simulink model "AuE8930_G2"  (R2023a)
settings: Solver=VariableStepAuto  StartTime=0  StopTime=2474  FixedStep=0.1  RelTol=1e-3
undefined symbols (not defined in the file): Af, alpha, Battery, Cd, eff_trans, EM_Omega_Max, EM_Torque_Max, frr, Ft_r_accl, Ft_r_decl, Fuel_Cell, g, Ki, Kp, mass, r_tire, ratio_fd, rho_air
libraries: fl_lib x16, nesl_utility x13, ee_lib x8, autolibshared x1, slpidlib x1, batteryecm_lib x1
settings Model: PacingRate=1000  Creator=akilp  LastModifiedBy=amrut
settings DebuggingCC: AlgebraicLoopMsg=none  UnconnectedInputMsg=warning  UnconnectedOutputMsg=warning  UnconnectedLineMsg=warning
settings ModelReferenceCC: EnableRefExpFcnMdlSchedulingChecks=on
settings SFSimCC: CustomCodeUndefinedFunction=UseInterfaceOnly
settings RTWCC: DLArmComputeVersion=19.05

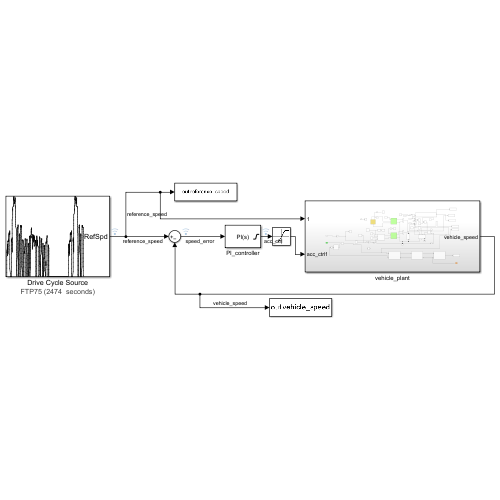
[thumbnail: Simulink's stored preview of the top-level diagram]
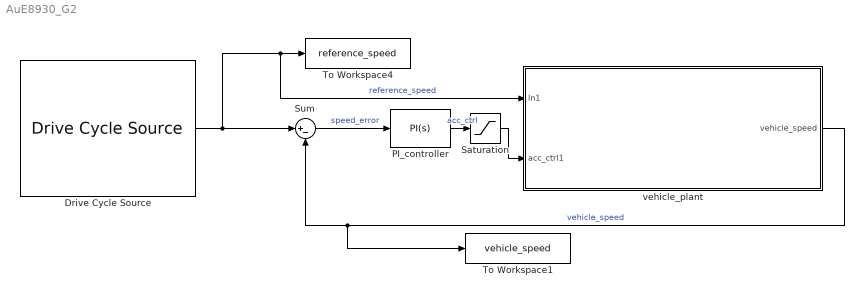
== system AuE8930_G2 ==
  Drive Cycle Source : autolibshared/Drive Cycle Source  cycleVar=FTP75  wsVar=high_trans_speed  fileVar=cycleFTP75.mat  tfinal="2474  seconds"  cycleRepeat=off  outAccPort=off  outGearPort=off  gearList=No gear data  t_wot1=5  xdot_woto=0  xdot_wot1=30  t_wot2=20  xdot_wot2=0  t_wotend=30  srcUnit=m/s  outUnit=m/s  srcAccUnit=m/s/s  outAccUnit=m/s^2  dt=0  aMode=1  faultOption=off  velBnd=2  velBndUnit=mph  inUnit=m/s  timeBnd=1  failOption=off  stopSim=off  maxFaultCnt=10  maxFaultTime=2  maxTotFaultTime=15  traceOption=off  dtTrace=1  traceWindow=10  lastDCname=FTP75  lastOutUnit=mph  lastDT=0  lastTB=1  lastSB=2  forceCalcBound=off
  "PI_controller " : slpidlib/PID Controller  Controller=PI  Form=Parallel  TimeDomain=Continuous-time  UseExternalTs=off  SampleTime=-1  IntegratorMethod=Forward Euler  FilterMethod=Forward Euler  ControllerParametersSource=internal  P=Kp  I=Ki  UseKiTs=off  D=0  N=100  UseFilter=on  TunerSelectOption=Transfer Function Based (PID Tuner App)  InitialConditionSource=internal  InitialConditionForIntegrator=0  InitialConditionForFilter=0  DifferentiatorICPrevScaledInput=0  ExternalReset=none  TrackingMode=off  Kt=1  LimitOutput=on  SatLimitsSource=internal  UpperSaturationLimit=1  LowerSaturationLimit=-1  LinearizeAsGain=on  AntiWindupMode=back-calculation  Kb=1  LimitIntegrator=off  UpperIntegratorSaturationLimit=inf  LowerIntegratorSaturationLimit=-inf  POutMin=[]  POutMax=[]  IOutMin=[]  IOutMax=[]  DOutMin=[]  DOutMax=[]  NOutMin=[]  NOutMax=[]  SumOutMin=[]  SumOutMax=[]  SaturationOutMin=[]  SaturationOutMax=[]  PParamMin=[]  PParamMax=[]  IParamMin=[]  IParamMax=[]  DParamMin=[]  DParamMax=[]  NParamMin=[]  NParamMax=[]  KbParamMin=[]  KbParamMax=[]  KtParamMin=[]  KtParamMax=[]  KbOutMin=[]  KbOutMax=[]  KtOutMin=[]  KtOutMax=[]  IntegratorOutMin=[]  IntegratorOutMax=[]  FilterOutMin=[]  FilterOutMax=[]  SumI1OutMin=[]  SumI1OutMax=[]  SumI2OutMin=[]  SumI2OutMax=[]  SumI3OutMin=[]  SumI3OutMax=[]  SumI4OutMin=[]  SumI4OutMax=[]  SumDOutMin=[]  SumDOutMax=[]  DifferentiatorOutMin=[]  DifferentiatorOutMax=[]  FilterDiffOutCoefMin=[]  FilterDiffOutCoefMax=[]  ReciprocalOutMin=[]  ReciprocalOutMax=[]  SumDenOutMin=[]  SumDenOutMax=[]  SumNumOutMin=[]  SumNumOutMax=[]  DivideOutMin=[]  DivideOutMax=[]  UdiffTsProdOutMin=[]  UdiffTsProdOutMax=[]  NTsProdOutMin=[]  NTsProdOutMax=[]  UintegralTsProdOutMin=[]  UintegralTsProdOutMax=[]  UngainTsProdOutMin=[]  UngainTsProdOutMax=[]  ClampingZeroOutDataTypeStr=Inherit: Inherit via back propagation  ClampingZeroOutMin=[]  ClampingZeroOutMax=[]  FilterDenConstantOutDataTypeStr=Inherit: Inherit via back propagation  FilterDenConstantOutMin=[]  FilterDenConstantOutMax=[]  PCopyOutDataTypeStr=Inherit: Inherit via back propagation  PCopyOutMin=[]  PCopyOutMax=[]  NCopyOutDataTypeStr=Inherit: Inherit via back propagation  NCopyOutMin=[]  NCopyOutMax=[]  IntegratorContinuousStateAttributes=''  IntegratorStateMustResolveToSignalObject=off  IntegratorRTWStateStorageClass=Auto  FilterContinuousStateAttributes=''  FilterStateMustResolveToSignalObject=off  FilterRTWStateStorageClass=Auto  ParallelPVariant=InternalParameters  IdealPVariant=Disabled  IVariant=InternalParameters  DVariant=Disabled  IntegratorVariant=Continuous  SatVariant=Enabled  AWVariant=BackCalculation  PCopyVariant=Disabled  TRVariant=Disabled  FdbkBlocksVariant=Forward  IdealPFdbkVariant=Disabled  SatFdbkVariant=Disabled  DerivativeFilterVariant=Disabled  NVariant=Disabled  NCopyVariant=Disabled_SignalSpec  FilterICVariant=Disabled  IntegratorICVariant=InternalICs  ExternalResetVariant=Disabled  TRSumVariant=Passthrough  SumFdbkVariant=Disabled  SumVariant=Sum_PI  TsampFilterVariant=InternalTs  TsampNgainVariant=Passthrough  TsampIntegralVariant=Disabled_SignalSpec  ExternalSaturationOutDataTypeStr=Inherit: Same as second input
  Saturation : Saturate  UpperLimit=100  LowerLimit=-100
  Sum : Sum  Inputs=|+-
  To Workspace1 : ToWorkspace  VariableName=vehicle_speed  SaveFormat=Timeseries  SampleTime=-1
  To Workspace4 : ToWorkspace  VariableName=reference_speed  SaveFormat=Timeseries  SampleTime=-1
  vehicle_plant : Subsystem
  wires:
  Sum/1 -> "PI_controller "/1  "speed_error"
  Drive Cycle Source/1 -> vehicle_plant/1(In1), To Workspace4/1, Sum/1  "reference_speed"
  vehicle_plant/1(vehicle_speed) -> To Workspace1/1, Sum/2  "vehicle_speed"
  "PI_controller "/1 -> Saturation/1  "acc_ctrl"
  Saturation/1 -> vehicle_plant/2(acc_ctrl1)

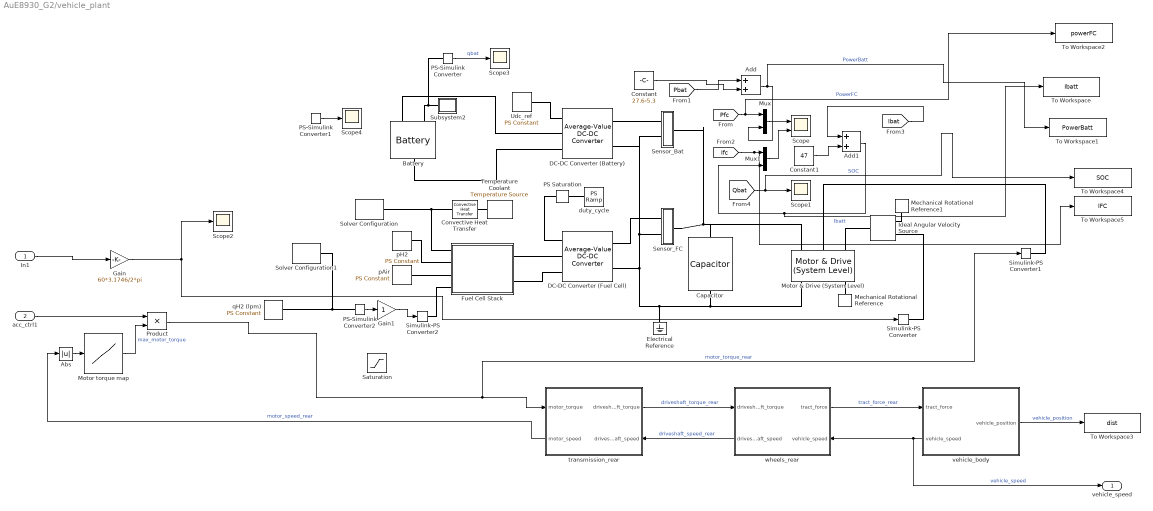
== system AuE8930_G2/vehicle_plant ==
  In1 : Inport
  acc_ctrl1 : Inport  Port=2
  Abs : Abs  SaturateOnIntegerOverflow=off
  Add : Sum
  Add1 : Sum
  Battery : batteryecm_lib/Battery  Vnom=Battery.Unom V  prm_dir=simscape.enum.battery.prm_dir.disabled  R1_dis=2 Ohm  R1_ch=2 Ohm  R1=Battery.Resistance Ohm  prm_AH=2  AH=Battery.Qnom hr*A  V1=Battery.U1 V  AH1=Battery.Q1 hr*A  prm_R2=1  R2=2000 Ohm  Tmeas=298.15 K  charge_measurement_port=simscape.enum.battery.enable.yes  prm_dyn=1  Rp1=0.005 Ohm  tau1=30 s  Rp2=0.005 Ohm  tau2=30 s  Rp3=0.005 Ohm  tau3=30 s  Rp4=0.005 Ohm  tau4=30 s  Rp5=0.005 Ohm  tau5=30 s  prm_fade=1  N_fade=100  AH_fade=45 hr*A  R1_fade=2.02 Ohm  R1_ch_fade=2.02 Ohm  V1_fade=10.35 V  prm_age=1  prm_age_OCV=1  OCV_age=0.9  SOC_age=60  Tmeas_age=298.15 K  delta_time_age_vec=[0] d  temperature_age_vec=[273] K  OCV_scaling_age=2.2134e6  OCV_offset_age=1.632e6  temp_exp_age=0.515833569 V  t_exp_age=0.75  Vnom_T2=12 V  R1_T2=2.2 Ohm  R1_T2_dis=2.2 Ohm  R1_T2_ch=2.2 Ohm  V1_T2=11.4 V  R2_T2=2200 Ohm  Rp1_T2=0.005 Ohm  tau1_T2=30 s  Rp2_T2=0.005 Ohm  tau2_T2=30 s  Rp3_T2=0.005 Ohm  tau3_T2=30 s  Rp4_T2=0.005 Ohm  tau4_T2=30 s  Rp5_T2=0.005 Ohm  tau5_T2=30 s  Tmeas2=273.15 K  thermal_port=simscape.enum.thermaleffects.omit  thermal_mass=30000 J/K  i_specify=off  i_priority=None  i=0 A  i_nominal_specify=off  i_nominal_unit=A  i_nominal_value=1  v_specify=on  v_priority=High  v=Battery.Uinit V  v_nominal_specify=off  v_nominal_unit=V  v_nominal_value=1  charge_specify=on  charge_priority=High  charge=Battery.Qnom hr*A  charge_nominal_specify=off  charge_nominal_unit=A*hr  charge_nominal_value=1  num_cycles_specify=off  num_cycles_priority=High  num_cycles=0  num_cycles_nominal_specify=off  num_cycles_nominal_unit=1  num_cycles_nominal_value=1  temperature_specify=off  temperature_priority=High  temperature=298.15 K  temperature_nominal_specify=off  temperature_nominal_unit=K  temperature_nominal_value=1
      settings: LogSimulationData=on  InternalSimscapePortConfiguration="{\"Bottom\":[],\"Left\":[{\"id\":\"p\",\"label\":\"+\",\"type\":\"foundation.electrical.electrical\"},{\"id\":\"q\",\"label\":\"q\",\"type\":\"output\"}],\"Right\":[{\"id\":\"n\",\"label\":\"-\",\"type\":\"foundation.electrical.electrical\"}],\"Top\":[]}"
  Capacitor : fl_lib/Electrical/Electrical Elements/Capacitor  c=5 mF  r=0.05 Ohm  g=0 1/Ohm  i_specify=off  i_priority=None  i=0 A  i_nominal_specify=off  i_nominal_unit=A  i_nominal_value=1  v_specify=off  v_priority=None  v=0 V  v_nominal_specify=off  v_nominal_unit=V  v_nominal_value=1  vc_specify=on  vc_priority=High  vc=500 V  vc_nominal_specify=off  vc_nominal_unit=V  vc_nominal_value=1
  Constant : Constant  Value=27.6-5.3
  Constant1 : Constant  Value=47
  Convective Heat Transfer : fl_lib/Thermal/Thermal Elements/Convective Heat Transfer  thermal_type=foundation.enum.constant_variable.constant  area=300 cm^2  heat_tr_coeff=75 W/(m^2 * K)  min_heat_tr_coeff=1e-3 W/(K*m^2)  T_specify=off  T_priority=None  T=0 K  T_nominal_specify=off  T_nominal_unit=K  T_nominal_value=1  Q_specify=off  Q_priority=None  Q=0 W  Q_nominal_specify=off  Q_nominal_unit=W  Q_nominal_value=1
  DC-DC Converter (Battery) : ee_lib/Semiconductors & Converters/Converters/Average-Value DC-DC Converter  control_option=ee.enum.converters.controlinput.voltage  converter_type=ee.enum.converters.dcdctype.boost  efficiency_option=ee.enum.converters.efficiency.constant  efficiency_fixed=100  i_vec=[0, 2, 5] A  efficiency_vec=[90, 95, 98]
      settings: LogSimulationData=on  InternalSimscapePortConfiguration="{\"Bottom\":[],\"Left\":[{\"id\":\"Vref\",\"label\":\"Vref\",\"type\":\"input\"},{\"id\":\"p1\",\"label\":\"1+\",\"type\":\"foundation.electrical.electrical\"},{\"id\":\"n1\",\"label\":\"1-\",\"type\":\"foundation.electrical.electrical\"}],\"Right\":[{\"id\":\"p2\",\"label\":\"2+\",\"type\":\"foundation.electrical.electrical\"},{\"id\":\"n2\",\"label\":\"2-\",\"type\":\"foundation.electrical.electrical\"}],\"Top\":[]}"
  DC-DC Converter (Fuel Cell) : ee_lib/Semiconductors & Converters/Converters/Average-Value DC-DC Converter  control_option=ee.enum.converters.controlinput.dutycycle  converter_type=ee.enum.converters.dcdctype.boost  efficiency_option=ee.enum.converters.efficiency.constant  efficiency_fixed=100  i_vec=[0, 2, 5] A  efficiency_vec=[90, 95, 98]
      settings: LogSimulationData=on  InternalSimscapePortConfiguration="{\"Bottom\":[],\"Left\":[{\"id\":\"DutyCycle\",\"label\":\"DutyCycle\",\"type\":\"input\"},{\"id\":\"p1\",\"label\":\"1+\",\"type\":\"foundation.electrical.electrical\"},{\"id\":\"n1\",\"label\":\"1-\",\"type\":\"foundation.electrical.electrical\"}],\"Right\":[{\"id\":\"p2\",\"label\":\"2+\",\"type\":\"foundation.electrical.electrical\"},{\"id\":\"n2\",\"label\":\"2-\",\"type\":\"foundation.electrical.electrical\"}],\"Top\":[]}"
  Electrical Reference : fl_lib/Electrical/Electrical Elements/Electrical Reference
  Fuel Cell Stack : Subsystem
  Gain : Gain  Gain=60*3.1746/2*pi
  Gain1 : Gain
  Ideal Angular Velocity Source : fl_lib/Mechanical/Mechanical Sources/Ideal Angular Velocity Source
  Mechanical Rotational Reference : fl_lib/Mechanical/Rotational Elements/Mechanical Rotational Reference
  Mechanical Rotational Reference1 : fl_lib/Mechanical/Rotational Elements/Mechanical Rotational Reference
  Motor & Drive (System Level) : ee_lib/Electromechanical/Motor & Drive (System Level)  torque_speed_param=ee.enum.electromech.envelope.torque_power  overtorque_param=ee.enum.electromech.overtorque.no  T_t=[.09, .08, .07, 0] N*m  T_t_intermittent=[.36, .32, .28, 0] N*m  T_t_2D=[.09, .09, .09; .08, .08, .08; .07, .07, .07; 0, 0, 0] N*m  T_t_intermittent_2D=[.36, .36, .36; .32, .32, .32; .28, .28, .28; 0, 0, 0] N*m  w_t=[0, 3750, 7500, 8000] rpm  vdc_t=[6, 12, 24] V  torque_max=Electric_Motor.Torque N*m  power_max=Electric_Motor.Power kW  torque_max_intermittent=0.4 N*m  power_max_intermittent=120 W  time_overtorque=30 s  time_recover=60 s  Tc=0.02 s  losses_param=1  eff=100  w_eff=3750 rpm  T_eff=0.08 N*m  Piron=0 W  Pbase=0 W  w_eff_vec=[-8000, -4000, 0, 4000, 8000] rpm  T_eff_vec=[0, .03, .06, .09] N*m  v_eff_vec=[100, 250, 400] V  losses_mat=[1.49, 1.67, 2.21, 3.1; .42, .69, 1.14, 2.03; .06, .24, .78, 1.68; .42, .69, 1.14, 2.03; 1.49, 1.67, 2.21, 3.1] W  efficiency_mat=[95, 95, 95, 95; 95, 95, 95, 95; 95, 95, 95, 95; 95, 95, 95, 95; 95, 95, 95, 95]  losses_mat_3D=ones(5, 4, 3) W  efficiency_mat_3D=95 * ones(5, 4, 3)  Res=0 Ohm  enable_fault=simscape.enum.onoff.off  fault_condition=1  fault_threshold=0.5  J=5e-6 kg*m^2  lam=1e-5 N*m/(rad/s)  speed0=0 rpm  faulted_specify=off  faulted_priority=None  faulted=0  faulted_nominal_specify=off  faulted_nominal_unit=1  faulted_nominal_value=1  torqueLimitContinuous_specify=off  torqueLimitContinuous_priority=None  torqueLimitContinuous=0 N*m  torqueLimitContinuous_nominal_specify=off  torqueLimitContinuous_nominal_unit=N*m  torqueLimitContinuous_nominal_value=1  alpha=3.93e-3 1/K  Tmeas=25 degC  Tmeas2=125 degC  losses_mat_T2=[1.49, 1.74, 2.49, 3.74; .42, .67, 1.42, 2.67; .06, .31, 1.06, 2.31; .42, .67, 1.42, 2.67; 1.49, 1.74, 2.49, 3.74] W  efficiency_mat_T2=[95, 95, 95, 95; 95, 95, 95, 95; 95, 95, 95, 95; 95, 95, 95, 95; 95, 95, 95, 95]  losses_mat_3D_T2=ones(5, 4, 3) W  efficiency_mat_3D_T2=95 * ones(5, 4, 3)  thermal_mass=100 J/K  initial_temperature=25 degC
  Motor torque map : Lookup_n-D  NumberOfTableDimensions=1  BreakpointsForDimension1=EM_Omega_Max  BreakpointsForDimension2=alpha  Table=EM_Torque_Max  ExtrapMethod=Clip  UseLastTableValue=on  InternalRulePriority=Speed  RndMeth=Simplest
  Mux : Mux  Inputs=2
  Mux1 : Mux  Inputs=2
  PS Saturation : fl_lib/Physical Signals/Nonlinear Operators/PS Saturation  upper_limit=0.95  lower_limit=0.15
  PS-Simulink Converter : nesl_utility/PS-Simulink Converter  PhysicalDomain=network_engine_domain  SubClassName=ps_output  LeftPortType=input  RightPortType=output  PseudoPeriodic=off  Frequencies=[]  VectorFormat=inherit  Unit=inherit  AffineConversion=off
  PS-Simulink Converter1 : nesl_utility/PS-Simulink Converter  PhysicalDomain=network_engine_domain  SubClassName=ps_output  LeftPortType=input  RightPortType=output  PseudoPeriodic=off  Frequencies=[]  VectorFormat=inherit  Unit=inherit  AffineConversion=off
  PS-Simulink Converter2 : nesl_utility/PS-Simulink Converter  PhysicalDomain=network_engine_domain  SubClassName=ps_output  LeftPortType=input  RightPortType=output  PseudoPeriodic=off  Frequencies=[]  VectorFormat=inherit  Unit=inherit  AffineConversion=off
  Product : Product
  Saturation : Saturate
  Scope : Scope  NumInputPorts=2
  Scope{1..4} (4 alike) : Scope
  Sensor_Bat : Subsystem
  Sensor_FC : Subsystem
  Simulink-PS Converter : nesl_utility/Simulink-PS Converter  PhysicalDomain=network_engine_domain  SubClassName=ps_input  LeftPortType=input  RightPortType=output  PseudoPeriodic=off  Frequencies=[]  NoiseDistribution=none  NoiseParameters=[]  Unit=rad/s  AffineConversion=off  FilteringAndDerivatives=filter  SimscapeFilterOrder=1  InputFilterTimeConstant=1  UdotUserProvided=0
  Simulink-PS Converter1 : nesl_utility/Simulink-PS Converter  PhysicalDomain=network_engine_domain  SubClassName=ps_input  LeftPortType=input  RightPortType=output  PseudoPeriodic=off  Frequencies=[]  NoiseDistribution=none  NoiseParameters=[]  Unit=N*m  AffineConversion=off  FilteringAndDerivatives=filter  SimscapeFilterOrder=1  InputFilterTimeConstant=1  UdotUserProvided=0
  Simulink-PS Converter2 : nesl_utility/Simulink-PS Converter  PhysicalDomain=network_engine_domain  SubClassName=ps_input  LeftPortType=input  RightPortType=output  PseudoPeriodic=off  Frequencies=[]  NoiseDistribution=none  NoiseParameters=[]  Unit=1  AffineConversion=off  FilteringAndDerivatives=provide  SimscapeFilterOrder=1  InputFilterTimeConstant=0.001  UdotUserProvided=0
  Solver Configuration : nesl_utility/Solver Configuration  PhysicalDomain=network_engine_domain  SubClassName=solver  LeftPortType=input  RightPortType=generic  Tones=[]  Harmonics=[]  SimulateNoise=off  Profile=off  UseLocalSampling=off  EnableSwitchedLinearOptims=on  FrequencyDomain=off  UseCCode=off  RelTol=0.001  AbsTol=1e-06  MinStep=1e-09  ToWorkspace=off  RevertToSquareIcSolve=off  NumHomotopyIterations=100  PhasorMode=off  PhasorModeNumHarmonics=1  ConsistencySolver=NEWTON_FTOL  IndexReductionMethod=DerivativeReplacement  DoDC=off  ResidualTolerance=1e-09  ConsistencyTolSource=GLOBAL  ConsistencyAbsTol=0.001  ConsistencyRelTol=0.001  ConsistencyTolFactor=0.001  UseLocalSolver=on  LocalSolverChoice=NE_BACKWARD_EULER_ADVANCER  ResolveIndetEquations=on  FunctionEvalNumThread=1  LocalSolverSampleTime=0.001  DoFixedCost=on  MaxNonlinIter=3  MaxModeIter=2  ComputeImpulses=off  ImpulseIterations=2  LinearAlgebra=auto  LinearAlgebraNumThread=0  EquationFormulation=NE_TIME_EF  DelaysMemoryBudget=1024  AutomaticFiltering=on  FilteringTimeConstant=0.001  PartitionStorageMethod=AS_NEEDED  PartitionMemoryBudget=1024  PartitionMethod=ROBUST
  Solver Configuration1 : nesl_utility/Solver Configuration  PhysicalDomain=network_engine_domain  SubClassName=solver  LeftPortType=input  RightPortType=generic  Tones=[]  Harmonics=[]  SimulateNoise=off  Profile=off  UseLocalSampling=off  EnableSwitchedLinearOptims=on  FrequencyDomain=off  UseCCode=off  RelTol=0.001  AbsTol=0.001  MinStep=1e-09  ToWorkspace=off  RevertToSquareIcSolve=off  NumHomotopyIterations=100  PhasorMode=off  PhasorModeNumHarmonics=1  ConsistencySolver=NEWTON_XTOL_AFTER_FTOL  IndexReductionMethod=DerivativeReplacement  DoDC=off  ResidualTolerance=1e-09  ConsistencyTolSource=GLOBAL  ConsistencyAbsTol=0.001  ConsistencyRelTol=0.001  ConsistencyTolFactor=0.001  UseLocalSolver=on  LocalSolverChoice=NE_PARTITIONING_ADVANCER  ResolveIndetEquations=on  FunctionEvalNumThread=1  LocalSolverSampleTime=0.001  DoFixedCost=on  MaxNonlinIter=3  MaxModeIter=2  ComputeImpulses=off  ImpulseIterations=2  LinearAlgebra=auto  LinearAlgebraNumThread=0  EquationFormulation=NE_TIME_EF  DelaysMemoryBudget=1024  AutomaticFiltering=on  FilteringTimeConstant=0.001  PartitionStorageMethod=AS_NEEDED  PartitionMemoryBudget=1024  PartitionMethod=ROBUST
  Subsystem2 : Subsystem
  Temperature Coolant : fl_lib/Thermal/Thermal Sources/Temperature Source  temperature=293.15 K
  To Workspace : ToWorkspace  VariableName=Ibatt  SaveFormat=Timeseries  SampleTime=-1
  To Workspace1 : ToWorkspace  VariableName=PowerBatt  SaveFormat=Timeseries  SampleTime=-1
  To Workspace2 : ToWorkspace  VariableName=powerFC  SaveFormat=Timeseries  SampleTime=-1
  To Workspace3 : ToWorkspace  VariableName=dist  SaveFormat=Timeseries  SampleTime=-1
  To Workspace4 : ToWorkspace  VariableName=SOC  SaveFormat=Timeseries  SampleTime=-1
  To Workspace5 : ToWorkspace  VariableName=IFC  SaveFormat=Timeseries  SampleTime=-1
  Udc_ref : fl_lib/Physical Signals/Sources/PS Constant  constant=480
  duty_cycle : fl_lib/Physical Signals/Sources/PS Ramp  slope=-0.8/60 1/s  start_time=0 s  initial_output=0.95
  pAir : fl_lib/Physical Signals/Sources/PS Constant  constant=1 bar
  pH2 : fl_lib/Physical Signals/Sources/PS Constant  constant=5.0 bar
  qH2 (lpm) : fl_lib/Physical Signals/Sources/PS Constant  constant=80 lpm
  transmission_rear : Subsystem
      settings: PortSchema="{\"entries\":[{\"content\":{\"sides\":[{\"content\":{\"connectorIds\":[\"In1\",\"Out2\"]},\"type\":\"ConnectorPlacement.EquallySpacedRectSide\",\"uuid\":\"9ce22768-c180-462f-8dee-6b9f8dff1999\"},{\"content\":{\"connectorIds\":[\"Out1\",\"In2\"],\"side\":\"RIGHT\"},\"type\":\"ConnectorPlacement.EquallySpacedRectSide\",\"uuid\":\"e4325ae3-643c-48c0-9eeb-31c7447b47db\"},{\"content\":{\"connectorIds\":[],\"side\":\"TOP\"},\"type\":\"ConnectorPlacement.EquallySpacedRectSide\",\"uuid\":\"152bd153-84b9-4199-b479-93a561dd7e82\"}]},\"type\":\"ConnectorPlacement.EquallySpacedConnector\",\"uuid\":\"8a72cfa2-d01f-44e6-be2e-c405844b3074\"}],\"packageUris\":[\"http://schema.mathworks.com/mf0/Connector/R2020b\"],\"version\":\"1.0\"}"
  vehicle_body : Subsystem
      settings: PortSchema="{\"entries\":[{\"content\":{\"sides\":[{\"content\":{\"connectorIds\":[\"In1\",\"Out2\"]},\"type\":\"ConnectorPlacement.EquallySpacedRectSide\",\"uuid\":\"9ce22768-c180-462f-8dee-6b9f8dff1999\"},{\"content\":{\"connectorIds\":[\"Out1\"],\"side\":\"RIGHT\"},\"type\":\"ConnectorPlacement.EquallySpacedRectSide\",\"uuid\":\"e4325ae3-643c-48c0-9eeb-31c7447b47db\"},{\"content\":{\"connectorIds\":[],\"side\":\"TOP\"},\"type\":\"ConnectorPlacement.EquallySpacedRectSide\",\"uuid\":\"152bd153-84b9-4199-b479-93a561dd7e82\"}]},\"type\":\"ConnectorPlacement.EquallySpacedConnector\",\"uuid\":\"8a72cfa2-d01f-44e6-be2e-c405844b3074\"}],\"packageUris\":[\"http://schema.mathworks.com/mf0/Connector/R2020b\"],\"version\":\"1.0\"}"
  wheels_rear : Subsystem
      settings: PortSchema="{\"entries\":[{\"content\":{\"sides\":[{\"content\":{\"connectorIds\":[\"In1\",\"Out2\"]},\"type\":\"ConnectorPlacement.EquallySpacedRectSide\",\"uuid\":\"9ce22768-c180-462f-8dee-6b9f8dff1999\"},{\"content\":{\"connectorIds\":[\"Out1\",\"In2\"],\"side\":\"RIGHT\"},\"type\":\"ConnectorPlacement.EquallySpacedRectSide\",\"uuid\":\"e4325ae3-643c-48c0-9eeb-31c7447b47db\"},{\"content\":{\"connectorIds\":[],\"side\":\"TOP\"},\"type\":\"ConnectorPlacement.EquallySpacedRectSide\",\"uuid\":\"152bd153-84b9-4199-b479-93a561dd7e82\"}]},\"type\":\"ConnectorPlacement.EquallySpacedConnector\",\"uuid\":\"8a72cfa2-d01f-44e6-be2e-c405844b3074\"}],\"packageUris\":[\"http://schema.mathworks.com/mf0/Connector/R2020b\"],\"version\":\"1.0\"}"
  vehicle_speed : Outport
  wires:
  vehicle_body/1(vehicle_position) -> To Workspace3/1  "vehicle_position"
  vehicle_body/2(vehicle_speed) -> vehicle_speed/1, wheels_rear/2(vehicle_speed)  "vehicle_speed"
  wheels_rear/2(driveshaft_speed) -> transmission_rear/2(driveshaft_speed)  "driveshaft_speed_rear"
  wheels_rear/1(tract_force) -> vehicle_body/1(tract_force)  "tract_force_rear"
  transmission_rear/1(driveshaft_torque) -> wheels_rear/1(driveshaft_torque)  "driveshaft_torque_rear"
  Product/1 -> Simulink-PS Converter1/1, transmission_rear/1(motor_torque)  "motor_torque_rear"
  transmission_rear/2(motor_speed) -> Abs/1  "motor_speed_rear"
  acc_ctrl1/1 -> Product/1
  Abs/1 -> Motor torque map/1
  Motor torque map/1 -> Product/2  "max_motor_torque"
  In1/1 -> Gain/1
  [Ifc] -> To Workspace5/1, Mux1/1
  Mux1/1 -> Scope/2
  Mux/1 -> Scope/1
  [Pfc] -> To Workspace2/1, Mux/1  "PowerFC"
  Gain/1 -> Simulink-PS Converter/1, Scope2/1
  [Pbat] -> Add/1
  Constant/1 -> Add/2
  Add/1 -> To Workspace1/1, Mux/2  "PowerBatt"
  [Ibat] -> Add1/1
  Add1/1 -> Mux1/2, To Workspace/1  "Ibatt"
  Constant1/1 -> Add1/2
  [Qbat] -> To Workspace4/1, Scope1/1  "SOC"
  PS-Simulink Converter/1 -> Scope3/1  "qbat"
  PS-Simulink Converter1/1 -> Scope4/1
  PS-Simulink Converter2/1 -> Gain1/1
  Gain1/1 -> Simulink-PS Converter2/1
  connections:
  Solver Configuration/RConn1 -- Convective Heat Transfer/LConn1 -- Fuel Cell Stack/LConn1
  Sensor_FC/RConn1 -- Capacitor/LConn1 -- Motor & Drive (System Level)/LConn1 -- Sensor_Bat/RConn1
  DC-DC Converter (Fuel Cell)/RConn2 -- DC-DC Converter (Battery)/RConn2 -- Sensor_Bat/LConn2 -- Sensor_FC/LConn2 -- Electrical Reference/LConn1 -- Motor & Drive (System Level)/RConn1 -- Capacitor/RConn1
  Mechanical Rotational Reference/LConn1 -- Motor & Drive (System Level)/RConn3
  DC-DC Converter (Fuel Cell)/RConn1 -- Sensor_FC/LConn1
  Battery/RConn1 -- DC-DC Converter (Battery)/LConn3
  DC-DC Converter (Fuel Cell)/LConn2 -- Fuel Cell Stack/RConn1
  DC-DC Converter (Battery)/LConn2 -- Battery/LConn1
  pAir/RConn1 -- Fuel Cell Stack/LConn3
  duty_cycle/RConn1 -- PS Saturation/LConn1
  PS Saturation/RConn1 -- DC-DC Converter (Fuel Cell)/LConn1
  Fuel Cell Stack/RConn2 -- DC-DC Converter (Fuel Cell)/LConn3
  Temperature Coolant/LConn1 -- Convective Heat Transfer/RConn1
  Mechanical Rotational Reference1/LConn1 -- Ideal Angular Velocity Source/RConn2
  DC-DC Converter (Battery)/RConn1 -- Sensor_Bat/LConn1
  Ideal Angular Velocity Source/LConn1 -- Motor & Drive (System Level)/LConn3
  Udc_ref/RConn1 -- DC-DC Converter (Battery)/LConn1
  Subsystem2/LConn1 -- PS-Simulink Converter/LConn1 -- Battery/LConn2
  pH2/RConn1 -- Fuel Cell Stack/LConn2
  Simulink-PS Converter1/RConn1 -- Motor & Drive (System Level)/LConn2
  Simulink-PS Converter/RConn1 -- Ideal Angular Velocity Source/RConn1
  Solver Configuration1/RConn1 -- qH2 (lpm)/RConn1 -- PS-Simulink Converter2/LConn1
  Simulink-PS Converter2/RConn1 -- Fuel Cell Stack/LConn4

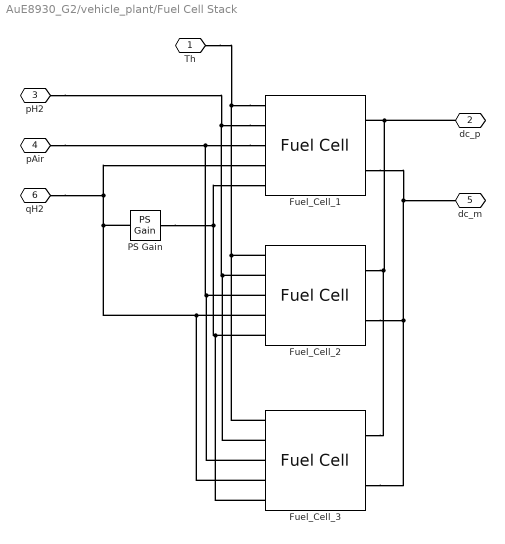
== system AuE8930_G2/vehicle_plant/Fuel Cell Stack ==
  Fuel_Cell_1 : ee_lib/Sources/Fuel Cell  model_fidelity=ee.enum.fuelcell.fidelity.detailed  Eoc=Fuel_Cell.OC_Voltage V  A=Fuel_Cell.Tafel_Slope V  ri=Fuel_Cell.Resistance Ohm  i0=Fuel_Cell.Exchange_Current A  i_lim=Fuel_Cell.Collapse_Current A  N_cell=65  number_unit=10  pH2_nom=Fuel_Cell.pH2_nom Pa  pO2_nom=Fuel_Cell.pAir_nom Pa  xH2=99  xO2=21  xW=1  dyn=ee.enum.include.no  Rd=0.005 Ohm  tau=10 s  Tnom=293.15 K  thermal_mass=30000 J/K  iFC_specify=off  iFC_priority=None  iFC=0 A  iFC_nominal_specify=off  iFC_nominal_unit=A  iFC_nominal_value=1  vFC_specify=off  vFC_priority=None  vFC=0 V  vFC_nominal_specify=off  vFC_nominal_unit=V  vFC_nominal_value=1  temperature_specify=off  temperature_priority=High  temperature=293 K  temperature_nominal_specify=off  temperature_nominal_unit=K  temperature_nominal_value=1
      settings: LogSimulationData=on  InternalSimscapePortConfiguration="{\"Bottom\":[],\"Left\":[{\"id\":\"H\",\"label\":\"H\",\"type\":\"foundation.thermal.thermal\"},{\"id\":\"pfuel\",\"label\":\"pfuel\",\"type\":\"input\"},{\"id\":\"pair\",\"label\":\"pair\",\"type\":\"input\"},{\"id\":\"qfuel\",\"label\":\"qfuel\",\"type\":\"input\"},{\"id\":\"qair\",\"label\":\"qair\",\"type\":\"input\"}],\"Right\":[{\"id\":\"p\",\"label\":\"+\",\"type\":\"foundation.electrical.electrical\"},{\"id\":\"n\",\"label\":\"-\",\"type\":\"foundation.electrical.electrical\"}],\"Top\":[]}"
  Fuel_Cell_2 : ee_lib/Sources/Fuel Cell  model_fidelity=ee.enum.fuelcell.fidelity.detailed  Eoc=Fuel_Cell.OC_Voltage V  A=Fuel_Cell.Tafel_Slope V  ri=Fuel_Cell.Resistance Ohm  i0=Fuel_Cell.Exchange_Current A  i_lim=Fuel_Cell.Collapse_Current A  N_cell=65  number_unit=10  pH2_nom=Fuel_Cell.pH2_nom Pa  pO2_nom=Fuel_Cell.pAir_nom Pa  xH2=99  xO2=21  xW=1  dyn=ee.enum.include.no  Rd=0.005 Ohm  tau=10 s  Tnom=293.15 K  thermal_mass=30000 J/K  iFC_specify=off  iFC_priority=None  iFC=0 A  iFC_nominal_specify=off  iFC_nominal_unit=A  iFC_nominal_value=1  vFC_specify=off  vFC_priority=None  vFC=0 V  vFC_nominal_specify=off  vFC_nominal_unit=V  vFC_nominal_value=1  temperature_specify=off  temperature_priority=High  temperature=293 K  temperature_nominal_specify=off  temperature_nominal_unit=K  temperature_nominal_value=1
      settings: LogSimulationData=on  InternalSimscapePortConfiguration="{\"Bottom\":[],\"Left\":[{\"id\":\"H\",\"label\":\"H\",\"type\":\"foundation.thermal.thermal\"},{\"id\":\"pfuel\",\"label\":\"pfuel\",\"type\":\"input\"},{\"id\":\"pair\",\"label\":\"pair\",\"type\":\"input\"},{\"id\":\"qfuel\",\"label\":\"qfuel\",\"type\":\"input\"},{\"id\":\"qair\",\"label\":\"qair\",\"type\":\"input\"}],\"Right\":[{\"id\":\"p\",\"label\":\"+\",\"type\":\"foundation.electrical.electrical\"},{\"id\":\"n\",\"label\":\"-\",\"type\":\"foundation.electrical.electrical\"}],\"Top\":[]}"
  Fuel_Cell_3 : ee_lib/Sources/Fuel Cell  model_fidelity=ee.enum.fuelcell.fidelity.detailed  Eoc=Fuel_Cell.OC_Voltage V  A=Fuel_Cell.Tafel_Slope V  ri=Fuel_Cell.Resistance Ohm  i0=Fuel_Cell.Exchange_Current A  i_lim=Fuel_Cell.Collapse_Current A  N_cell=65  number_unit=10  pH2_nom=Fuel_Cell.pH2_nom Pa  pO2_nom=Fuel_Cell.pAir_nom Pa  xH2=99  xO2=21  xW=1  dyn=ee.enum.include.no  Rd=0.005 Ohm  tau=10 s  Tnom=293.15 K  thermal_mass=30000 J/K  iFC_specify=off  iFC_priority=None  iFC=0 A  iFC_nominal_specify=off  iFC_nominal_unit=A  iFC_nominal_value=1  vFC_specify=off  vFC_priority=None  vFC=0 V  vFC_nominal_specify=off  vFC_nominal_unit=V  vFC_nominal_value=1  temperature_specify=off  temperature_priority=High  temperature=293 K  temperature_nominal_specify=off  temperature_nominal_unit=K  temperature_nominal_value=1
      settings: LogSimulationData=on  InternalSimscapePortConfiguration="{\"Bottom\":[],\"Left\":[{\"id\":\"H\",\"label\":\"H\",\"type\":\"foundation.thermal.thermal\"},{\"id\":\"pfuel\",\"label\":\"pfuel\",\"type\":\"input\"},{\"id\":\"pair\",\"label\":\"pair\",\"type\":\"input\"},{\"id\":\"qfuel\",\"label\":\"qfuel\",\"type\":\"input\"},{\"id\":\"qair\",\"label\":\"qair\",\"type\":\"input\"}],\"Right\":[{\"id\":\"p\",\"label\":\"+\",\"type\":\"foundation.electrical.electrical\"},{\"id\":\"n\",\"label\":\"-\",\"type\":\"foundation.electrical.electrical\"}],\"Top\":[]}"
  PS Gain : fl_lib/Physical Signals/Functions/PS Gain  gain=3
  Th : PMIOPort  Side=Left
  dc_p : PMIOPort  Port=2  Side=Right
  pH2 : PMIOPort  Port=3  Side=Left
  pAir : PMIOPort  Port=4  Side=Left
  dc_m : PMIOPort  Port=5  Side=Right
  qH2 : PMIOPort  Port=6  Side=Left
  connections:
  Fuel_Cell_1/RConn2 -- Fuel_Cell_3/RConn2 -- Fuel_Cell_2/RConn2 -- dc_m/RConn1
  Fuel_Cell_1/RConn1 -- dc_p/RConn1 -- Fuel_Cell_3/RConn1 -- Fuel_Cell_2/RConn1
  Fuel_Cell_1/LConn2 -- pH2/RConn1 -- Fuel_Cell_3/LConn2 -- Fuel_Cell_2/LConn2
  PS Gain/RConn1 -- Fuel_Cell_3/LConn5 -- Fuel_Cell_2/LConn5 -- Fuel_Cell_1/LConn5
  Fuel_Cell_3/LConn4 -- Fuel_Cell_2/LConn4 -- PS Gain/LConn1 -- qH2/RConn1 -- Fuel_Cell_1/LConn4
  Fuel_Cell_1/LConn3 -- pAir/RConn1 -- Fuel_Cell_3/LConn3 -- Fuel_Cell_2/LConn3
  Fuel_Cell_1/LConn1 -- Th/RConn1 -- Fuel_Cell_2/LConn1 -- Fuel_Cell_3/LConn1

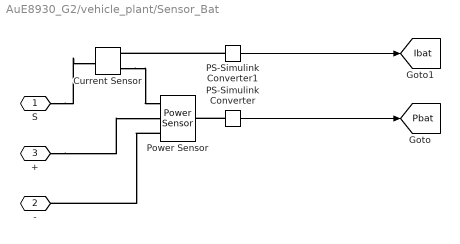
== system AuE8930_G2/vehicle_plant/Sensor_Bat ==
  Current Sensor : fl_lib/Electrical/Electrical Sensors/Current Sensor
  PS-Simulink Converter : nesl_utility/PS-Simulink Converter  PhysicalDomain=network_engine_domain  SubClassName=ps_output  LeftPortType=input  RightPortType=output  PseudoPeriodic=off  Frequencies=[]  VectorFormat=1-D array  Unit=kW  AffineConversion=off
  PS-Simulink Converter1 : nesl_utility/PS-Simulink Converter  PhysicalDomain=network_engine_domain  SubClassName=ps_output  LeftPortType=input  RightPortType=output  PseudoPeriodic=off  Frequencies=[]  VectorFormat=1-D array  Unit=A  AffineConversion=off
  Power Sensor : ee_lib/Sensors & Transducers/Power Sensor  measurement_type=1  averaging_period=1e-4 s
  S : PMIOPort  Side=Left
  - : PMIOPort  Port=2  Side=Left
  + : PMIOPort  Port=3  Side=Right
  tag scope: Ibat=global, Pbat=global
  wires:
  PS-Simulink Converter/1 -> [Pbat]
  PS-Simulink Converter1/1 -> [Ibat]
  connections:
  +/RConn1 -- Power Sensor/LConn2
  Power Sensor/LConn3 -- -/RConn1
  PS-Simulink Converter/LConn1 -- Power Sensor/RConn1
  Current Sensor/RConn2 -- Power Sensor/LConn1
  S/RConn1 -- Current Sensor/LConn1
  PS-Simulink Converter1/LConn1 -- Current Sensor/RConn1

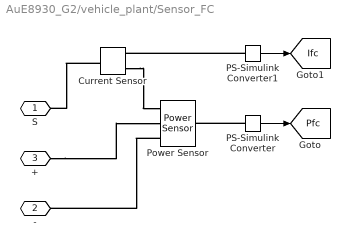
== system AuE8930_G2/vehicle_plant/Sensor_FC ==
  Current Sensor : fl_lib/Electrical/Electrical Sensors/Current Sensor
  PS-Simulink Converter : nesl_utility/PS-Simulink Converter  PhysicalDomain=network_engine_domain  SubClassName=ps_output  LeftPortType=input  RightPortType=output  PseudoPeriodic=off  Frequencies=[]  VectorFormat=1-D array  Unit=kW  AffineConversion=off
  PS-Simulink Converter1 : nesl_utility/PS-Simulink Converter  PhysicalDomain=network_engine_domain  SubClassName=ps_output  LeftPortType=input  RightPortType=output  PseudoPeriodic=off  Frequencies=[]  VectorFormat=1-D array  Unit=A  AffineConversion=off
  Power Sensor : ee_lib/Sensors & Transducers/Power Sensor  measurement_type=1  averaging_period=1e-4 s
  S : PMIOPort  Side=Left
  - : PMIOPort  Port=2  Side=Left
  + : PMIOPort  Port=3  Side=Right
  tag scope: Ifc=global, Pfc=global
  wires:
  PS-Simulink Converter/1 -> [Pfc]
  PS-Simulink Converter1/1 -> [Ifc]
  connections:
  +/RConn1 -- Power Sensor/LConn2
  Power Sensor/LConn3 -- -/RConn1
  PS-Simulink Converter/LConn1 -- Power Sensor/RConn1
  PS-Simulink Converter1/LConn1 -- Current Sensor/RConn1
  Current Sensor/LConn1 -- S/RConn1
  Current Sensor/RConn2 -- Power Sensor/LConn1

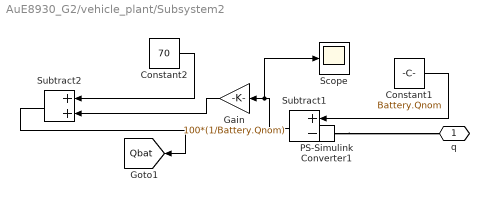
== system AuE8930_G2/vehicle_plant/Subsystem2 ==
  Constant1 : Constant  Value=Battery.Qnom
  Constant2 : Constant  Value=70
  Gain : Gain  Gain=100*(1/Battery.Qnom)
  PS-Simulink Converter1 : nesl_utility/PS-Simulink Converter  PhysicalDomain=network_engine_domain  SubClassName=ps_output  LeftPortType=input  RightPortType=output  PseudoPeriodic=off  Frequencies=[]  VectorFormat=1-D array  Unit=A*hr  AffineConversion=off
  Scope : Scope
  Subtract1 : Sum  Inputs=+-
  Subtract2 : Sum
  q : PMIOPort  Side=Left
  tag scope: Qbat=global
  wires:
  Subtract1/1 -> Scope/1, Gain/1
  PS-Simulink Converter1/1 -> Subtract1/2
  Constant1/1 -> Subtract1/1
  Constant2/1 -> Subtract2/1
  Gain/1 -> Subtract2/2
  Subtract2/1 -> [Qbat]
  connections:
  PS-Simulink Converter1/LConn1 -- q/RConn1

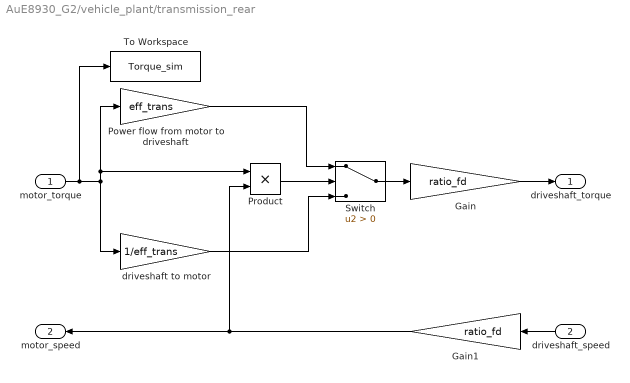
== system AuE8930_G2/vehicle_plant/transmission_rear ==
  motor_torque : Inport
  driveshaft_speed : Inport  Port=2
  Gain : Gain  Gain=ratio_fd
  Gain1 : Gain  Gain=ratio_fd
  Power flow from motor to driveshaft : Gain  Gain=eff_trans
  Product : Product
  Switch : Switch  Criteria=u2 > Threshold  SaturateOnIntegerOverflow=off  InputSameDT=off
  To Workspace : ToWorkspace  VariableName=Torque_sim  SampleTime=-1
  driveshaft to motor : Gain  Gain=1/eff_trans
  driveshaft_torque : Outport
  motor_speed : Outport  Port=2
  wires:
  motor_torque/1 -> To Workspace/1, Power flow from motor to driveshaft/1, Product/1, driveshaft to motor/1
  Switch/1 -> Gain/1
  driveshaft to motor/1 -> Switch/3
  Power flow from motor to driveshaft/1 -> Switch/1
  Gain/1 -> driveshaft_torque/1
  Gain1/1 -> Product/2, motor_speed/1
  driveshaft_speed/1 -> Gain1/1
  Product/1 -> Switch/2

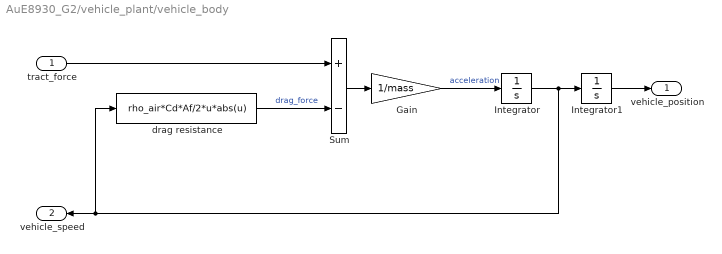
== system AuE8930_G2/vehicle_plant/vehicle_body ==
  tract_force : Inport
  Gain : Gain  Gain=1/mass
  Integrator : Integrator
  Integrator1 : Integrator
  Sum : Sum  Inputs=+-
  drag resistance : Fcn  Expr=rho_air*Cd*Af/2*u*abs(u)
  vehicle_position : Outport
  vehicle_speed : Outport  Port=2
  wires:
  tract_force/1 -> Sum/1
  Integrator/1 -> drag resistance/1, vehicle_speed/1, Integrator1/1
  Gain/1 -> Integrator/1  "acceleration"
  Integrator1/1 -> vehicle_position/1
  Sum/1 -> Gain/1
  drag resistance/1 -> Sum/2  "drag_force"

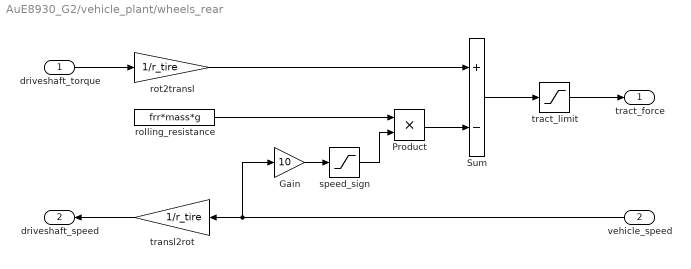
== system AuE8930_G2/vehicle_plant/wheels_rear ==
  driveshaft_torque : Inport
  vehicle_speed : Inport  Port=2
  Gain : Gain  Gain=10
  Product : Product
  Sum : Sum  Inputs=+-
  rolling_resistance : Constant  Value=frr*mass*g
  rot2transl : Gain  Gain=1/r_tire
  speed_sign : Saturate  UpperLimit=1  LowerLimit=-1  LinearizeAsGain=off
  tract_limit : Saturate  UpperLimit=Ft_r_accl  LowerLimit=Ft_r_decl
  transl2rot : Gain  Gain=1/r_tire
  tract_force : Outport
  driveshaft_speed : Outport  Port=2
  wires:
  driveshaft_torque/1 -> rot2transl/1
  Sum/1 -> tract_limit/1
  transl2rot/1 -> driveshaft_speed/1
  vehicle_speed/1 -> Gain/1, transl2rot/1
  rot2transl/1 -> Sum/1
  rolling_resistance/1 -> Product/1
  Product/1 -> Sum/2
  speed_sign/1 -> Product/2
  tract_limit/1 -> tract_force/1
  Gain/1 -> speed_sign/1
